simulink model "chargingHubTwin"  (R2026a)
settings: Solver=FixedStepDiscrete  StartTime=0  StopTime=23  FixedStep=1
settings Model: Creator=Gourav Nanak  LastModifiedBy=Gourav Nanak

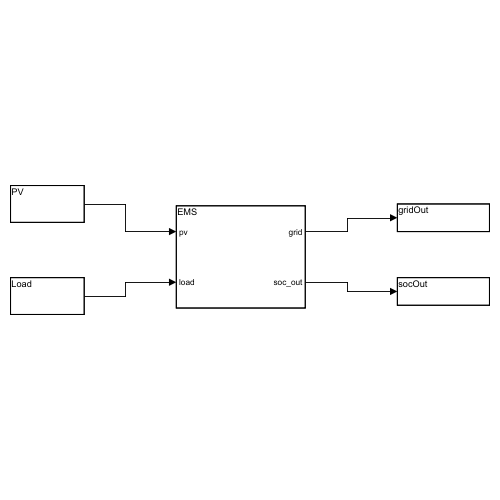
[thumbnail: Simulink's stored preview of the top-level diagram]
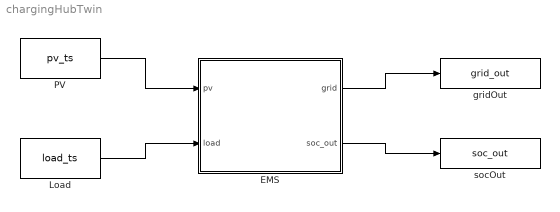
== system chargingHubTwin ==
  EMS : MATLAB Function  TreatAsAtomicUnit=on
  Load : FromWorkspace  VariableName=load_ts  Interpolate=off  OutputAfterFinalValue=Holding final value
  PV : FromWorkspace  VariableName=pv_ts  Interpolate=off  OutputAfterFinalValue=Holding final value
  gridOut : ToWorkspace  VariableName=grid_out  SampleTime=-1
  socOut : ToWorkspace  VariableName=soc_out  SampleTime=-1
  wires:
  PV/1 -> EMS/1(pv)
  Load/1 -> EMS/2(load)
  EMS/1(grid) -> gridOut/1
  EMS/2(soc_out) -> socOut/1

== matlab function chargingHubTwin/EMS ==
  data: pv input; grid output; load input; soc_out output
function [grid, soc_out] = EMS(pv, load)
persistent soc
usable = 27.000000; eta = 0.959166; pmax = 15.000000;
if isempty(soc); soc = usable*0.5; end
a = min(pv, load); res = load - a; sur = pv - a;
if sur > 0
    room = (usable - soc)/eta; c = min([sur, pmax, room]);
    if c < 0; c = 0; end
    soc = soc + c*eta; sur = sur - c;
end
g = 0;
if res > 0
    if soc > 0
        dis = min([res, pmax, soc*eta]);
        if dis < 0; dis = 0; end
        soc = soc - dis/eta; res = res - dis;
    end
    g = max(res, 0);
end
grid = g; soc_out = soc;
